simulink model "Quadcopter_FE_and_FTC_Sim"  (R2021a)
settings: Solver=VariableStepAuto  StartTime=0.0  StopTime=10.0  RelTol=1e-3
values from neighbouring files (symbols this model uses):
  A1_bar = [A1 E;zeros(3,6) zeros(3,3)]    [Quadcopter_Fault_Parameters_and_Flags.m]
  A2_bar = [A2 E;zeros(3,6) zeros(3,3)]    [Quadcopter_Fault_Parameters_and_Flags.m]
  A3_bar = [A3 E;zeros(3,6) zeros(3,3)]    [Quadcopter_Fault_Parameters_and_Flags.m]
  A4_bar = [A4 E;zeros(3,6) zeros(3,3)]    [Quadcopter_Fault_Parameters_and_Flags.m]
  B_bar = [B;zeros(3,3)]    [Quadcopter_Fault_Parameters_and_Flags.m]
  d = 0.0301    [Quadcopter_Fault_Parameters_and_Flags.m]
  Delta_q = [1 1 1 1;1 -1 -1 1;1 1 -1 -1;-1 1 -1 1]    [Quadcopter_Fault_Parameters_and_Flags.m]
  g = 9.8066    [Quadcopter_Fault_Parameters_and_Flags.m]
  Jrz = 2.029 * 10^(-5)    (= 2.029e-05)    [Quadcopter_Fault_Parameters_and_Flags.m]
  Jx = 0.0022    [Quadcopter_Fault_Parameters_and_Flags.m]
  Jy = 0.0029    [Quadcopter_Fault_Parameters_and_Flags.m]
  Jz = 0.0048    [Quadcopter_Fault_Parameters_and_Flags.m]
  K_D_kesi = diag([0.08,0.08,0.22])    [Quadcopter_Fault_Parameters_and_Flags.m]
  K_D_omega = diag([0.2,0.2,0.5])    [Quadcopter_Fault_Parameters_and_Flags.m]
  K_P_kesi = diag([0.18,0.18,052])    [Quadcopter_Fault_Parameters_and_Flags.m]
  K_P_omega = diag([1.5,1.5,2])    [Quadcopter_Fault_Parameters_and_Flags.m]
  kesi_d = [0 0 0]'    [Quadcopter_Fault_Parameters_and_Flags.m]
  kesi_dot_d = [0 0 0]'    [Quadcopter_Fault_Parameters_and_Flags.m]
  l = 0.1785    [Quadcopter_Fault_Parameters_and_Flags.m]
  LPI1_bar = (P^-1)*M    [Quadcopter_Fault_Parameters_and_Flags.m]
  LPI2_bar = (P^-1)*M    [Quadcopter_Fault_Parameters_and_Flags.m]
  LPI3_bar = (P^-1)*M    [Quadcopter_Fault_Parameters_and_Flags.m]
  LPI4_bar = (P^-1)*M    [Quadcopter_Fault_Parameters_and_Flags.m]
  m = 0.4080    (= 0.408)    [Quadcopter_Fault_Parameters_and_Flags.m]
  O_d = [0 0 0]'    [Quadcopter_Fault_Parameters_and_Flags.m]
  Omega_d = [0 0 0]'    [Quadcopter_Fault_Parameters_and_Flags.m]
  Omega_M = 475    [Quadcopter_Fault_Parameters_and_Flags.m]
  Phi_dot_init = 0    [Quadcopter_Fault_Parameters_and_Flags.m]
  Phi_init = 0    [Quadcopter_Fault_Parameters_and_Flags.m]
  Psi_dot_init = 0    [Quadcopter_Fault_Parameters_and_Flags.m]
  Psi_init = 0    [Quadcopter_Fault_Parameters_and_Flags.m]
  Theta_dot_init = 0    [Quadcopter_Fault_Parameters_and_Flags.m]
  Theta_init = 0    [Quadcopter_Fault_Parameters_and_Flags.m]
  x_dot_init = 0    [Quadcopter_Fault_Parameters_and_Flags.m]
  x_init = 0    [Quadcopter_Fault_Parameters_and_Flags.m]
  y_dot_init = 0    [Quadcopter_Fault_Parameters_and_Flags.m]
  y_init = 0    [Quadcopter_Fault_Parameters_and_Flags.m]
  z_dot_init = 0    [Quadcopter_Fault_Parameters_and_Flags.m]
  z_init = 0    [Quadcopter_Fault_Parameters_and_Flags.m]
settings Model: Creator=kiankhaneghahi  LastModifiedBy=kiankhaneghahi

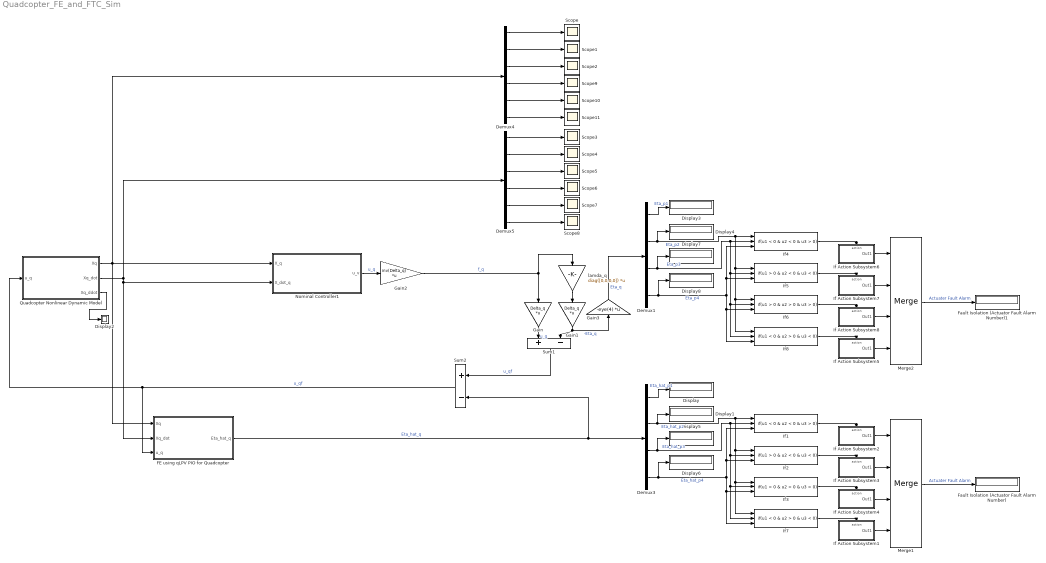
== system Quadcopter_FE_and_FTC_Sim ==
  Demux1 : Demux
  Demux3 : Demux
  Demux4 : Demux  Outputs=6
  Demux5 : Demux  Outputs=6
  Display{,1..8} (9 alike) : Display
  FE using qLPV PIO for Quadcopter : Subsystem
  Fault Isolation (Actuator Fault Alarm Number) : Display
  Fault Isolation (Actuator Fault Alarm Number)1 : Display
  Gain : Gain  Gain=Delta_q  Multiplication=Matrix(K*u)
  Gain1 : Gain  Gain=Delta_q  Multiplication=Matrix(K*u)
  Gain2 : Gain  Gain=inv(Delta_q)  Multiplication=Matrix(K*u)
  Gain3 : Gain  Gain=-eye(4)  Multiplication=Matrix(K*u)
  If Action Subsystem1 : Subsystem  TreatAsAtomicUnit=on
  If Action Subsystem2 : Subsystem  TreatAsAtomicUnit=on
  If Action Subsystem3 : Subsystem  TreatAsAtomicUnit=on
  If Action Subsystem4 : Subsystem  TreatAsAtomicUnit=on
  If Action Subsystem5 : Subsystem  TreatAsAtomicUnit=on
  If Action Subsystem6 : Subsystem  TreatAsAtomicUnit=on
  If Action Subsystem7 : Subsystem  TreatAsAtomicUnit=on
  If Action Subsystem8 : Subsystem  TreatAsAtomicUnit=on
  If1 : If  NumInputs=3  IfExpression=u1 < 0 & u2 < 0 & u3 > 0  ShowElse=off
  If2 : If  NumInputs=3  IfExpression=u1 > 0 & u2 < 0 & u3 < 0  ShowElse=off
  If3 : If  NumInputs=3  IfExpression=u1 > 0 & u2 > 0 & u3 > 0  ShowElse=off
  If4 : If  NumInputs=3  IfExpression=u1 < 0 & u2 < 0 & u3 > 0  ShowElse=off
  If5 : If  NumInputs=3  IfExpression=u1 > 0 & u2 < 0 & u3 < 0  ShowElse=off
  If6 : If  NumInputs=3  IfExpression=u1 > 0 & u2 > 0 & u3 > 0  ShowElse=off
  If7 : If  NumInputs=3  IfExpression=u1 < 0 & u2 > 0 & u3 < 0  ShowElse=off
  If8 : If  NumInputs=3  IfExpression=u1 < 0 & u2 > 0 & u3 < 0  ShowElse=off
  Merge1 : Merge  Inputs=4
  Merge2 : Merge  Inputs=4
  Nominal Controller1 : Subsystem
  Quadcopter Nonlinear Dynamic Model : Subsystem
  Scope{,1..11} (12 alike) : Scope
  Sum1 : Sum  Inputs=+-
  Sum2 : Sum  Inputs=+-
  lamda_q : Gain  Gain=diag([0,0,0,0])  Multiplication=Matrix(K*u)
  wires:
  If Action Subsystem3/1(Out1) -> Merge1/2
  lamda_q/1 -> Gain1/1
  Demux3/2 -> If7/1, If3/1, If2/1, If1/1, Display1/1  "Eta_hat_p2"
  Demux5/2 -> Scope4/1
  Demux3/3 -> If3/2, If7/2, If2/2, If1/2, Display5/1  "Eta_hat_p3"
  If2/1 -> If Action Subsystem3/Action
  Gain/1 -> Sum1/1  "u_q"
  Quadcopter Nonlinear Dynamic Model/2(Xq_dot) -> Demux5/1, Nominal Controller1/2(X_dot_q), FE using qLPV PIO for Quadcopter/2(Xq_dot)
  Merge1/1 -> Fault Isolation (Actuator Fault Alarm Number)/1  "Actuater Fault Alarm"
  If Action Subsystem4/1(Out1) -> Merge1/3
  If1/1 -> If Action Subsystem2/Action
  Demux4/1 -> Scope/1
  Nominal Controller1/1(u_v) -> Gain2/1  "u_q"
  Quadcopter Nonlinear Dynamic Model/1(Xq) -> Nominal Controller1/1(X_q), Demux4/1, FE using qLPV PIO for Quadcopter/1(Xq)
  Demux4/3 -> Scope2/1
  Demux4/2 -> Scope1/1
  Quadcopter Nonlinear Dynamic Model/3(Xq_ddot) -> Display2/1
  Gain2/1 -> Gain/1, lamda_q/1  "f_q"
  If Action Subsystem2/1(Out1) -> Merge1/1
  If3/1 -> If Action Subsystem4/Action
  Demux5/1 -> Scope3/1
  FE using qLPV PIO for Quadcopter/1(Eta_hat_q) -> Sum2/2, Demux3/1  "Eta_hat_q"
  Demux5/3 -> Scope5/1
  Sum2/1 -> Quadcopter Nonlinear Dynamic Model/1("u_q "), FE using qLPV PIO for Quadcopter/3(u_q)  "u_qf"
  Gain1/1 -> Sum1/2, Gain3/1  "-Eta_q"
  Gain3/1 -> Demux1/1  "Eta_q"
  Demux5/4 -> Scope6/1
  Demux5/5 -> Scope7/1
  Demux5/6 -> Scope8/1
  Demux4/5 -> Scope10/1
  Demux4/4 -> Scope9/1
  Demux4/6 -> Scope11/1
  Demux3/1 -> Display/1  "Eta_hat_p1"
  Demux3/4 -> If7/3, If3/3, If2/3, If1/3, Display6/1  "Eta_hat_p4"
  If Action Subsystem1/1(Out1) -> Merge1/4
  If7/1 -> If Action Subsystem1/Action
  Merge2/1 -> Fault Isolation (Actuator Fault Alarm Number)1/1  "Actuater Fault Alarm"
  If Action Subsystem8/1(Out1) -> Merge2/3
  If6/1 -> If Action Subsystem8/Action
  Demux1/1 -> Display3/1  "Eta_p1"
  If Action Subsystem7/1(Out1) -> Merge2/2
  If Action Subsystem6/1(Out1) -> Merge2/1
  If4/1 -> If Action Subsystem6/Action
  Demux1/3 -> If6/2, If8/2, If5/2, If4/2, Display7/1  "Eta_p3"
  Demux1/4 -> If8/3, If6/3, If5/3, If4/3, Display8/1  "Eta_p4"
  If5/1 -> If Action Subsystem7/Action
  Demux1/2 -> If8/1, If6/1, If5/1, If4/1, Display4/1  "Eta_p2"
  If8/1 -> If Action Subsystem5/Action
  If Action Subsystem5/1(Out1) -> Merge2/4
  Sum1/1 -> Sum2/1  "u_qf"

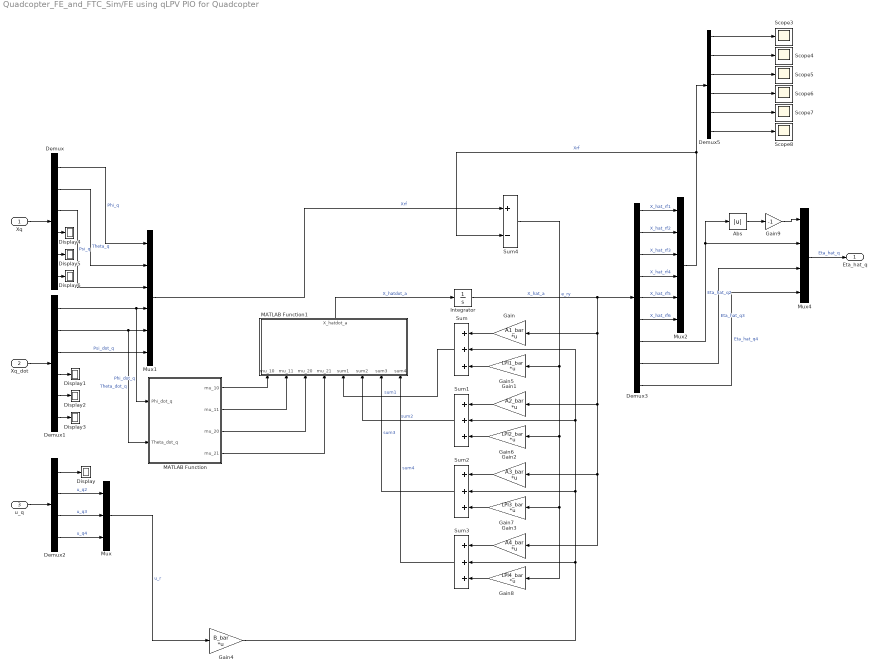
== system Quadcopter_FE_and_FTC_Sim/FE using qLPV PIO for Quadcopter ==
  Xq : Inport
  Xq_dot : Inport  Port=2
  u_q : Inport  Port=3
  Abs : Abs
  Demux : Demux  Outputs=6
  Demux1 : Demux  Outputs=6
  Demux2 : Demux
  Demux3 : Demux  Outputs=9
  Demux5 : Demux  Outputs=6
  Display{,1..6} (7 alike) : Display
  Gain : Gain  Gain=A1_bar  Multiplication=Matrix(K*u)
  Gain1 : Gain  Gain=A2_bar  Multiplication=Matrix(K*u)
  Gain2 : Gain  Gain=A3_bar  Multiplication=Matrix(K*u)
  Gain3 : Gain  Gain=A4_bar  Multiplication=Matrix(K*u)
  Gain4 : Gain  Gain=B_bar  Multiplication=Matrix(K*u)
  Gain5 : Gain  Gain=LPI1_bar  Multiplication=Matrix(K*u)
  Gain6 : Gain  Gain=LPI2_bar  Multiplication=Matrix(K*u)
  Gain7 : Gain  Gain=LPI3_bar  Multiplication=Matrix(K*u)
  Gain8 : Gain  Gain=LPI4_bar  Multiplication=Matrix(K*u)
  Gain9 : Gain  Gain=-1
  Integrator : Integrator
  MATLAB Function : MATLAB Function  TreatAsAtomicUnit=on
  MATLAB Function1 : MATLAB Function  TreatAsAtomicUnit=on
  Mux : Mux  Inputs=3
  Mux1 : Mux  Inputs=6
  Mux2 : Mux  Inputs=6
  Mux4 : Mux
  Scope{3..8} (6 alike) : Scope
  Sum{,1..3} (4 alike) : Sum  Inputs=+++
  Sum4 : Sum  Inputs=+-
  Eta_hat_q : Outport
  wires:
  Xq/1 -> Demux/1
  Xq_dot/1 -> Demux1/1
  u_q/1 -> Demux2/1
  Demux2/3 -> Mux/2  "u_q3"
  Demux2/2 -> Mux/1  "u_q2"
  Demux2/4 -> Mux/3  "u_q4"
  Mux/1 -> Gain4/1  "u_r"
  Demux/1 -> Mux1/1  "Phi_q"
  Demux/2 -> Mux1/2  "Theta_q"
  Demux/3 -> Mux1/3  "Psi_q"
  Demux1/1 -> MATLAB Function/1(Phi_dot_q), Mux1/4  "Phi_dot_q"
  Demux1/2 -> MATLAB Function/2(Theta_dot_q), Mux1/5  "Theta_dot_q"
  Demux1/3 -> Mux1/6  "Psi_dot_q"
  Mux1/1 -> Sum4/1  "Xrf"
  MATLAB Function1/1(X_hatdot_a) -> Integrator/1  "X_hatdot_a"
  Integrator/1 -> Gain3/1, Gain2/1, Gain1/1, Gain/1, Demux3/1  "X_hat_a"
  Gain/1 -> Sum/1
  Gain1/1 -> Sum1/1
  Gain2/1 -> Sum2/1
  Gain3/1 -> Sum3/1
  Gain4/1 -> Sum/2, Sum1/2, Sum2/2, Sum3/2
  Gain7/1 -> Sum2/3
  Gain5/1 -> Sum/3
  Gain6/1 -> Sum1/3
  Gain8/1 -> Sum3/3
  Demux3/1 -> Mux2/1  "X_hat_rf1"
  Demux3/2 -> Mux2/2  "X_hat_rf2"
  Demux3/3 -> Mux2/3  "X_hat_rf3"
  Demux3/4 -> Mux2/4  "X_hat_rf4"
  Demux3/5 -> Mux2/5  "X_hat_rf5"
  Demux3/6 -> Mux2/6  "X_hat_rf6"
  Demux3/7 -> Abs/1, Mux4/2  "Eta_hat_q2"
  Demux3/8 -> Mux4/3  "Eta_hat_q3"
  Demux3/9 -> Mux4/4  "Eta_hat_q4"
  Mux2/1 -> Demux5/1, Sum4/2  "Xrf"
  Sum4/1 -> Gain8/1, Gain7/1, Gain6/1, Gain5/1  "e_ry"
  Mux4/1 -> Eta_hat_q/1  "Eta_hat_q"
  Abs/1 -> Gain9/1
  Gain9/1 -> Mux4/1
  MATLAB Function/1(mu_10) -> MATLAB Function1/1(mu_10)
  MATLAB Function/2(mu_11) -> MATLAB Function1/2(mu_11)
  MATLAB Function/3(mu_20) -> MATLAB Function1/3(mu_20)
  MATLAB Function/4(mu_21) -> MATLAB Function1/4(mu_21)
  Sum/1 -> MATLAB Function1/5(sum1)  "sum1"
  Sum1/1 -> MATLAB Function1/6(sum2)  "sum2"
  Sum2/1 -> MATLAB Function1/7(sum3)  "sum3"
  Sum3/1 -> MATLAB Function1/8(sum4)  "sum4"
  Demux2/1 -> Display/1
  Demux1/4 -> Display1/1
  Demux1/5 -> Display2/1
  Demux1/6 -> Display3/1
  Demux/4 -> Display4/1
  Demux/5 -> Display5/1
  Demux/6 -> Display6/1
  Demux5/4 -> Scope6/1
  Demux5/1 -> Scope3/1
  Demux5/6 -> Scope8/1
  Demux5/2 -> Scope4/1
  Demux5/3 -> Scope5/1
  Demux5/5 -> Scope7/1

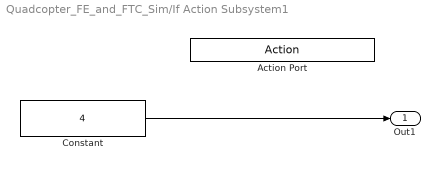
== system Quadcopter_FE_and_FTC_Sim/If Action Subsystem1 ==
  Action Port : ActionPort  ActionPortLabel=if(u1 < 0 & u2 > 0 & u3 < 0)
  Constant : Constant  Value=4
  Out1 : Outport
  wires:
  Constant/1 -> Out1/1

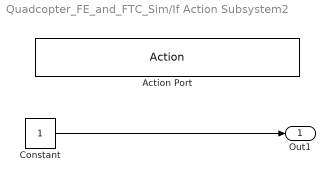
== system Quadcopter_FE_and_FTC_Sim/If Action Subsystem2 ==
  Action Port : ActionPort  ActionPortLabel=if(u1 < 0 & u2 < 0 & u3 > 0)
  Constant : Constant
  Out1 : Outport
  wires:
  Constant/1 -> Out1/1

== system Quadcopter_FE_and_FTC_Sim/If Action Subsystem3 ==
  Action Port : ActionPort  ActionPortLabel=if(u1 > 0 & u2 < 0 & u3 < 0)
  Constant : Constant  Value=2
  Out1 : Outport
  wires:
  Constant/1 -> Out1/1

== system Quadcopter_FE_and_FTC_Sim/If Action Subsystem4 ==
  Action Port : ActionPort  ActionPortLabel=if(u1 > 0 & u2 > 0 & u3 > 0)
  Constant : Constant  Value=3
  Out1 : Outport
  wires:
  Constant/1 -> Out1/1

== system Quadcopter_FE_and_FTC_Sim/If Action Subsystem5 ==
  Action Port : ActionPort  ActionPortLabel=if(u1 < 0 & u2 > 0 & u3 < 0)
  Constant : Constant  Value=4
  Out1 : Outport
  wires:
  Constant/1 -> Out1/1

== system Quadcopter_FE_and_FTC_Sim/If Action Subsystem6 ==
  Action Port : ActionPort  ActionPortLabel=if(u1 < 0 & u2 < 0 & u3 > 0)
  Constant : Constant
  Out1 : Outport
  wires:
  Constant/1 -> Out1/1

== system Quadcopter_FE_and_FTC_Sim/If Action Subsystem7 ==
  Action Port : ActionPort  ActionPortLabel=if(u1 > 0 & u2 < 0 & u3 < 0)
  Constant : Constant  Value=2
  Out1 : Outport
  wires:
  Constant/1 -> Out1/1

== system Quadcopter_FE_and_FTC_Sim/If Action Subsystem8 ==
  Action Port : ActionPort  ActionPortLabel=if(u1 > 0 & u2 > 0 & u3 > 0)
  Constant : Constant  Value=3
  Out1 : Outport
  wires:
  Constant/1 -> Out1/1

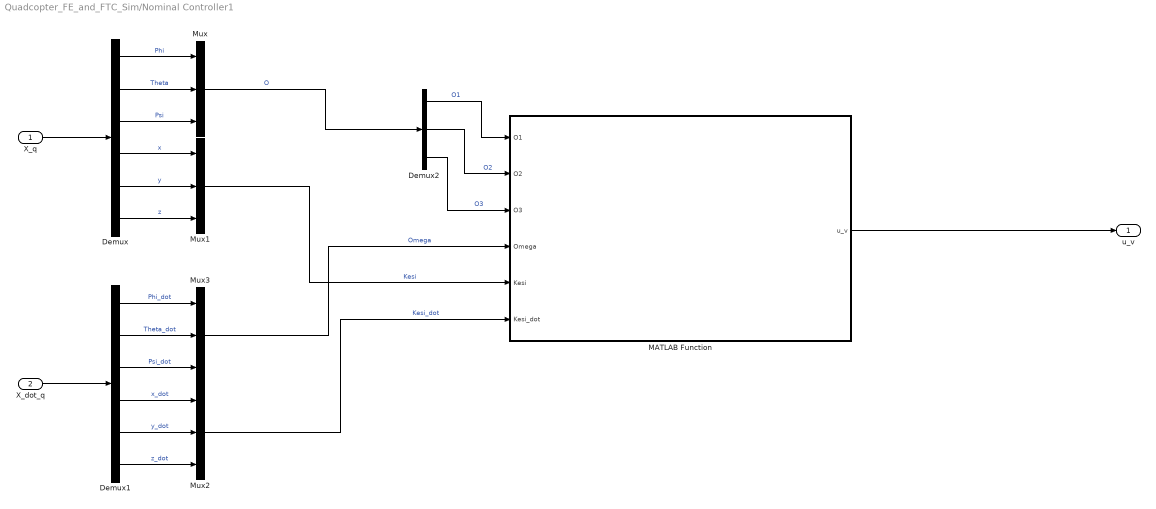
== system Quadcopter_FE_and_FTC_Sim/Nominal Controller1 ==
  X_q : Inport
  X_dot_q : Inport  Port=2
  Demux : Demux  Outputs=6
  Demux1 : Demux  Outputs=6
  Demux2 : Demux  Outputs=3
  MATLAB Function : MATLAB Function  TreatAsAtomicUnit=on
  Mux{,1..3} (4 alike) : Mux  Inputs=3
  u_v : Outport
  wires:
  X_q/1 -> Demux/1
  X_dot_q/1 -> Demux1/1
  Demux/3 -> Mux/3  "Psi"
  Demux/2 -> Mux/2  "Theta"
  Demux/1 -> Mux/1  "Phi"
  Demux/4 -> Mux1/1  "x"
  Demux/5 -> Mux1/2  "y"
  Demux/6 -> Mux1/3  "z"
  Demux1/4 -> Mux2/1  "x_dot"
  Demux1/5 -> Mux2/2  "y_dot"
  Demux1/6 -> Mux2/3  "z_dot"
  MATLAB Function/1(u_v) -> u_v/1
  Demux1/1 -> Mux3/1  "Phi_dot"
  Demux1/2 -> Mux3/2  "Theta_dot"
  Demux1/3 -> Mux3/3  "Psi_dot"
  Mux1/1 -> MATLAB Function/5(Kesi)  "Kesi"
  Mux2/1 -> MATLAB Function/6(Kesi_dot)  "Kesi_dot"
  Mux/1 -> Demux2/1  "O"
  Demux2/1 -> MATLAB Function/1(O1)  "O1"
  Demux2/2 -> MATLAB Function/2(O2)  "O2"
  Demux2/3 -> MATLAB Function/3(O3)  "O3"
  Mux3/1 -> MATLAB Function/4(Omega)  "Omega"

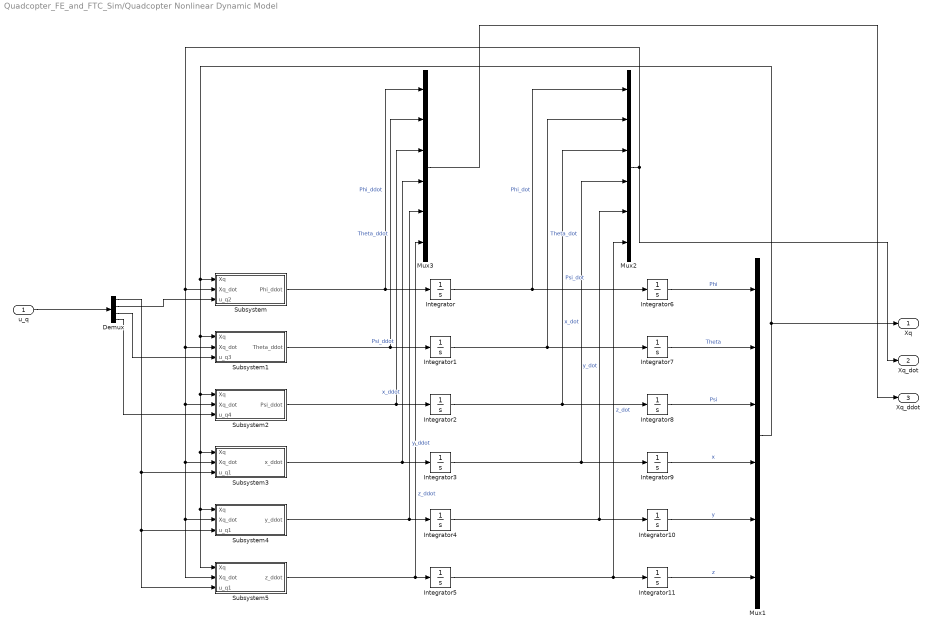
== system Quadcopter_FE_and_FTC_Sim/Quadcopter Nonlinear Dynamic Model ==
  "u_q " : Inport
  Demux : Demux
  Integrator : Integrator  InitialCondition=Phi_dot_init
  Integrator1 : Integrator  InitialCondition=Theta_dot_init
  Integrator10 : Integrator  InitialCondition=y_init
  Integrator11 : Integrator  InitialCondition=z_init
  Integrator2 : Integrator  InitialCondition=Psi_dot_init
  Integrator3 : Integrator  InitialCondition=x_dot_init
  Integrator4 : Integrator  InitialCondition=y_dot_init
  Integrator5 : Integrator  InitialCondition=z_dot_init
  Integrator6 : Integrator  InitialCondition=Phi_init
  Integrator7 : Integrator  InitialCondition=Theta_init
  Integrator8 : Integrator  InitialCondition=Psi_init
  Integrator9 : Integrator  InitialCondition=x_init
  Mux1 : Mux  Inputs=6
  Mux2 : Mux  Inputs=6
  Mux3 : Mux  Inputs=6
  Subsystem : Subsystem
  Subsystem1 : Subsystem
  Subsystem2 : Subsystem
  Subsystem3 : Subsystem
  Subsystem4 : Subsystem
  Subsystem5 : Subsystem
  Xq : Outport
  Xq_dot : Outport  Port=2
  Xq_ddot : Outport  Port=3
  wires:
  Integrator/1 -> Integrator6/1, Mux2/1  "Phi_dot"
  Integrator1/1 -> Mux2/2, Integrator7/1  "Theta_dot"
  Integrator2/1 -> Mux2/3, Integrator8/1  "Psi_dot"
  Integrator3/1 -> Mux2/4, Integrator9/1  "x_dot"
  Integrator4/1 -> Mux2/5, Integrator10/1  "y_dot"
  Integrator5/1 -> Mux2/6, Integrator11/1  "z_dot"
  Subsystem/1(Phi_ddot) -> Mux3/1, Integrator/1  "Phi_ddot"
  Subsystem5/1(z_ddot) -> Mux3/6, Integrator5/1  "z_ddot"
  Subsystem4/1(y_ddot) -> Mux3/5, Integrator4/1  "y_ddot"
  Subsystem3/1(x_ddot) -> Mux3/4, Integrator3/1  "x_ddot"
  Subsystem2/1(Psi_ddot) -> Mux3/3, Integrator2/1  "Psi_ddot"
  Subsystem1/1(Theta_ddot) -> Mux3/2, Integrator1/1  "Theta_ddot"
  "u_q "/1 -> Demux/1
  Demux/2 -> Subsystem/3(u_q2)
  Demux/3 -> Subsystem1/3(u_q3)
  Demux/4 -> Subsystem2/3(u_q4)
  Demux/1 -> Subsystem5/3(u_q1), Subsystem4/3(u_q1), Subsystem3/3(u_q1)
  Integrator6/1 -> Mux1/1  "Phi"
  Integrator7/1 -> Mux1/2  "Theta"
  Integrator8/1 -> Mux1/3  "Psi"
  Integrator9/1 -> Mux1/4  "x"
  Integrator10/1 -> Mux1/5  "y"
  Integrator11/1 -> Mux1/6  "z"
  Mux1/1 -> Subsystem5/1(Xq), Subsystem4/1(Xq), Subsystem3/1(Xq), Subsystem2/1(Xq), Subsystem1/1(Xq), Subsystem/1(Xq), Xq/1
  Mux2/1 -> Subsystem1/2(Xq_dot), Subsystem2/2(Xq_dot), Subsystem5/2(Xq_dot), Subsystem4/2(Xq_dot), Subsystem3/2(Xq_dot), Subsystem/2(Xq_dot), Xq_dot/1
  Mux3/1 -> Xq_ddot/1

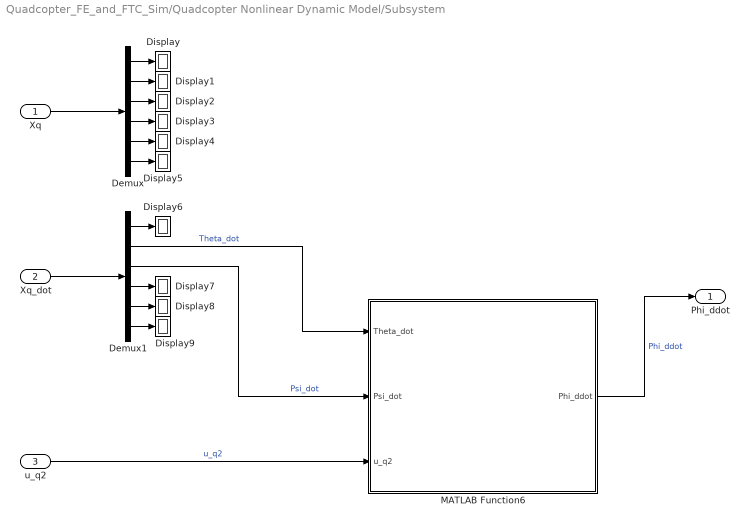
== system Quadcopter_FE_and_FTC_Sim/Quadcopter Nonlinear Dynamic Model/Subsystem ==
  Xq : Inport
  Xq_dot : Inport  Port=2
  u_q2 : Inport  Port=3
  Demux : Demux  Outputs=6
  Demux1 : Demux  Outputs=6
  Display{,1..9} (10 alike) : Display
  MATLAB Function6 : MATLAB Function  TreatAsAtomicUnit=on
  Phi_ddot : Outport
  wires:
  Xq/1 -> Demux/1
  Xq_dot/1 -> Demux1/1
  Demux1/2 -> MATLAB Function6/1(Theta_dot)  "Theta_dot"
  Demux1/3 -> MATLAB Function6/2(Psi_dot)  "Psi_dot"
  u_q2/1 -> MATLAB Function6/3(u_q2)  "u_q2"
  MATLAB Function6/1(Phi_ddot) -> Phi_ddot/1  "Phi_ddot"
  Demux/1 -> Display/1
  Demux/2 -> Display1/1
  Demux/3 -> Display2/1
  Demux/4 -> Display3/1
  Demux/5 -> Display4/1
  Demux/6 -> Display5/1
  Demux1/1 -> Display6/1
  Demux1/4 -> Display7/1
  Demux1/5 -> Display8/1
  Demux1/6 -> Display9/1

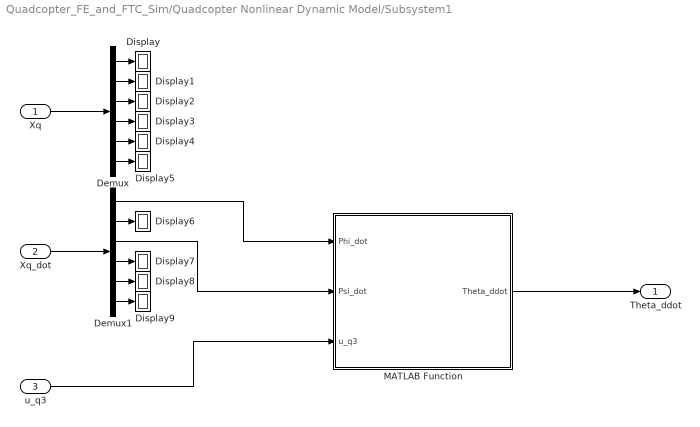
== system Quadcopter_FE_and_FTC_Sim/Quadcopter Nonlinear Dynamic Model/Subsystem1 ==
  Xq : Inport
  Xq_dot : Inport  Port=2
  u_q3 : Inport  Port=3
  Demux : Demux  Outputs=6
  Demux1 : Demux  Outputs=6
  Display{,1..9} (10 alike) : Display
  MATLAB Function : MATLAB Function  TreatAsAtomicUnit=on
  Theta_ddot : Outport
  wires:
  Xq/1 -> Demux/1
  Xq_dot/1 -> Demux1/1
  MATLAB Function/1(Theta_ddot) -> Theta_ddot/1
  u_q3/1 -> MATLAB Function/3(u_q3)
  Demux1/1 -> MATLAB Function/1(Phi_dot)
  Demux1/3 -> MATLAB Function/2(Psi_dot)
  Demux/1 -> Display/1
  Demux/2 -> Display1/1
  Demux/3 -> Display2/1
  Demux/4 -> Display3/1
  Demux/5 -> Display4/1
  Demux/6 -> Display5/1
  Demux1/2 -> Display6/1
  Demux1/4 -> Display7/1
  Demux1/5 -> Display8/1
  Demux1/6 -> Display9/1

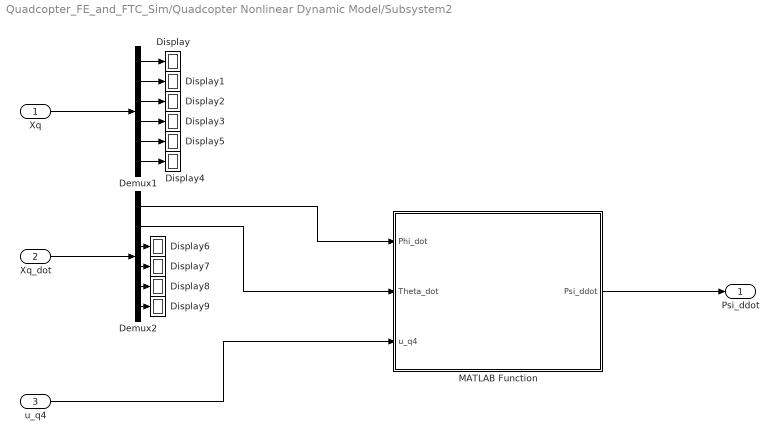
== system Quadcopter_FE_and_FTC_Sim/Quadcopter Nonlinear Dynamic Model/Subsystem2 ==
  Xq : Inport
  Xq_dot : Inport  Port=2
  u_q4 : Inport  Port=3
  Demux1 : Demux  Outputs=6
  Demux2 : Demux  Outputs=6
  Display{,1..9} (10 alike) : Display
  MATLAB Function : MATLAB Function  TreatAsAtomicUnit=on
  Psi_ddot : Outport
  wires:
  Xq/1 -> Demux1/1
  Xq_dot/1 -> Demux2/1
  MATLAB Function/1(Psi_ddot) -> Psi_ddot/1
  u_q4/1 -> MATLAB Function/3(u_q4)
  Demux2/1 -> MATLAB Function/1(Phi_dot)
  Demux2/2 -> MATLAB Function/2(Theta_dot)
  Demux1/1 -> Display/1
  Demux1/2 -> Display1/1
  Demux1/3 -> Display2/1
  Demux1/4 -> Display3/1
  Demux1/5 -> Display5/1
  Demux1/6 -> Display4/1
  Demux2/3 -> Display6/1
  Demux2/4 -> Display7/1
  Demux2/5 -> Display8/1
  Demux2/6 -> Display9/1

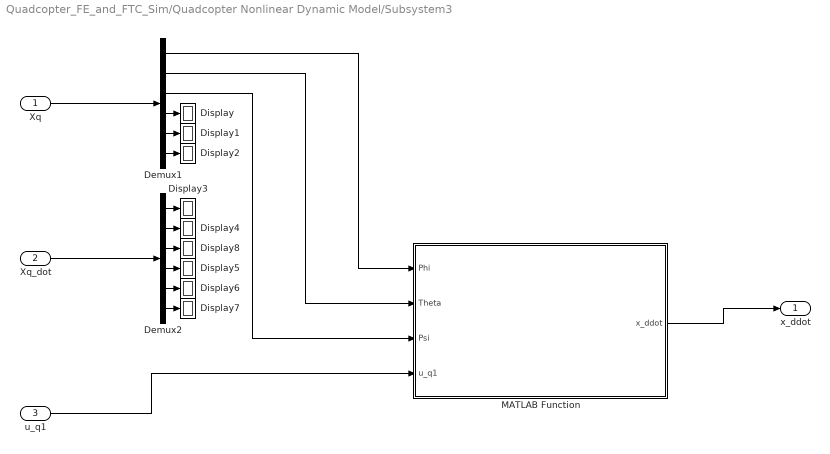
== system Quadcopter_FE_and_FTC_Sim/Quadcopter Nonlinear Dynamic Model/Subsystem3 ==
  Xq : Inport
  Xq_dot : Inport  Port=2
  u_q1 : Inport  Port=3
  Demux1 : Demux  Outputs=6
  Demux2 : Demux  Outputs=6
  Display{,1..8} (9 alike) : Display
  MATLAB Function : MATLAB Function  TreatAsAtomicUnit=on
  x_ddot : Outport
  wires:
  Xq/1 -> Demux1/1
  Xq_dot/1 -> Demux2/1
  MATLAB Function/1(x_ddot) -> x_ddot/1
  u_q1/1 -> MATLAB Function/4(u_q1)
  Demux1/1 -> MATLAB Function/1(Phi)
  Demux1/2 -> MATLAB Function/2(Theta)
  Demux1/3 -> MATLAB Function/3(Psi)
  Demux1/4 -> Display/1
  Demux1/5 -> Display1/1
  Demux1/6 -> Display2/1
  Demux2/1 -> Display3/1
  Demux2/2 -> Display4/1
  Demux2/3 -> Display8/1
  Demux2/4 -> Display5/1
  Demux2/5 -> Display6/1
  Demux2/6 -> Display7/1

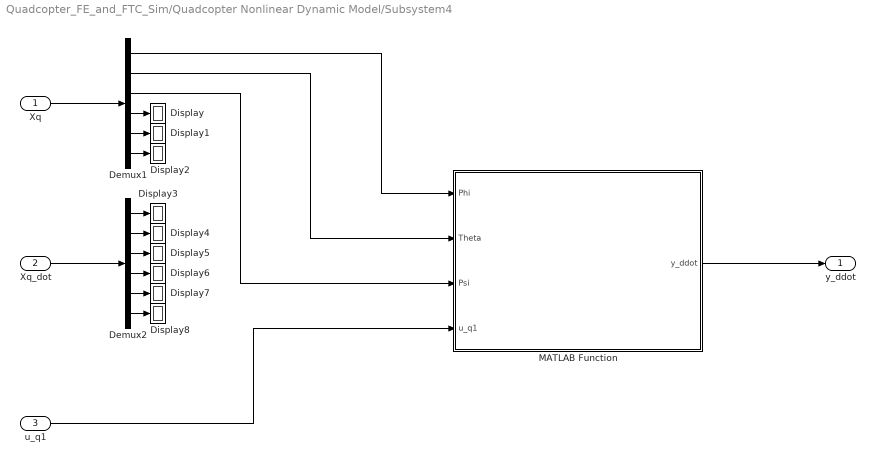
== system Quadcopter_FE_and_FTC_Sim/Quadcopter Nonlinear Dynamic Model/Subsystem4 ==
  Xq : Inport
  Xq_dot : Inport  Port=2
  u_q1 : Inport  Port=3
  Demux1 : Demux  Outputs=6
  Demux2 : Demux  Outputs=6
  Display{,1..8} (9 alike) : Display
  MATLAB Function : MATLAB Function  TreatAsAtomicUnit=on
  y_ddot : Outport
  wires:
  MATLAB Function/1(y_ddot) -> y_ddot/1
  Xq_dot/1 -> Demux2/1
  Xq/1 -> Demux1/1
  u_q1/1 -> MATLAB Function/4(u_q1)
  Demux1/1 -> MATLAB Function/1(Phi)
  Demux1/2 -> MATLAB Function/2(Theta)
  Demux1/3 -> MATLAB Function/3(Psi)
  Demux1/4 -> Display/1
  Demux1/5 -> Display1/1
  Demux1/6 -> Display2/1
  Demux2/1 -> Display3/1
  Demux2/2 -> Display4/1
  Demux2/3 -> Display5/1
  Demux2/4 -> Display6/1
  Demux2/5 -> Display7/1
  Demux2/6 -> Display8/1

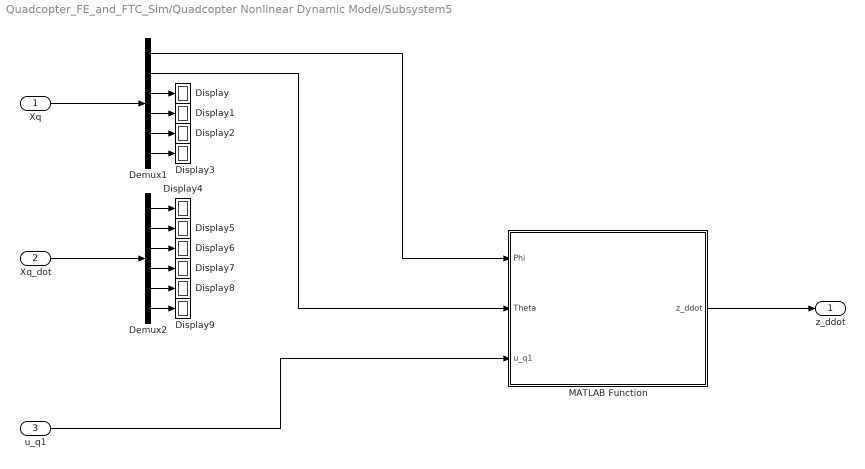
== system Quadcopter_FE_and_FTC_Sim/Quadcopter Nonlinear Dynamic Model/Subsystem5 ==
  Xq : Inport
  Xq_dot : Inport  Port=2
  u_q1 : Inport  Port=3
  Demux1 : Demux  Outputs=6
  Demux2 : Demux  Outputs=6
  Display{,1..9} (10 alike) : Display
  MATLAB Function : MATLAB Function  TreatAsAtomicUnit=on
  z_ddot : Outport
  wires:
  Xq/1 -> Demux1/1
  Xq_dot/1 -> Demux2/1
  MATLAB Function/1(z_ddot) -> z_ddot/1
  u_q1/1 -> MATLAB Function/3(u_q1)
  Demux1/1 -> MATLAB Function/1(Phi)
  Demux1/2 -> MATLAB Function/2(Theta)
  Demux1/3 -> Display/1
  Demux1/4 -> Display1/1
  Demux1/5 -> Display2/1
  Demux1/6 -> Display3/1
  Demux2/1 -> Display4/1
  Demux2/2 -> Display5/1
  Demux2/3 -> Display6/1
  Demux2/4 -> Display7/1
  Demux2/5 -> Display8/1
  Demux2/6 -> Display9/1

== matlab function Quadcopter_FE_and_FTC_Sim/FE using qLPV PIO for Quadcopter/MATLAB Function ==
  data: Phi_dot_q input; mu_10 output; Theta_dot_q input; mu_11 output; mu_20 output; mu_21 output
function [mu_10,mu_11,mu_20,mu_21] = fcn(Phi_dot_q, Theta_dot_q)
mu_10 = (pi-2*Phi_dot_q)/(2*pi);
mu_11 = 1-mu_10;
mu_20 = (pi-2*Theta_dot_q)/(2*pi);
mu_21 = 1-mu_20;

== matlab function Quadcopter_FE_and_FTC_Sim/FE using qLPV PIO for Quadcopter/MATLAB Function1 ==
  data: mu_10 input; X_hatdot_a output; mu_11 input; mu_20 input; mu_21 input; sum1 input; sum2 input; sum3 input; sum4 input
function X_hatdot_a = fcn(mu_10, mu_11, mu_20, mu_21, sum1, sum2, sum3, sum4)
ro_1 = mu_10 * mu_20;
ro_2 = mu_10 * mu_21;
ro_3 = mu_11 * mu_20;
ro_4 = mu_11 * mu_21;
X_hatdot_a = ro_1*sum1 + ro_2*sum2 + ro_3*sum3 + ro_4*sum4;

== matlab function Quadcopter_FE_and_FTC_Sim/Quadcopter Nonlinear Dynamic Model/Subsystem/MATLAB Function6 ==
  data: Theta_dot input; Phi_ddot output; Psi_dot input; u_q2 input; Jx parameter; Jy parameter; Jz parameter; Jrz parameter; Omega_M parameter; l parameter
function Phi_ddot = fcn(Theta_dot, Psi_dot, u_q2, Jx, Jy, Jz, Jrz, Omega_M, l)

Phi_ddot = Theta_dot*Psi_dot*((Jy-Jz)/Jx)-(Jrz/Jx)*Theta_dot*Omega_M+(l/Jx)*u_q2;

== matlab function Quadcopter_FE_and_FTC_Sim/Quadcopter Nonlinear Dynamic Model/Subsystem1/MATLAB Function ==
  data: Phi_dot input; Psi_dot input; u_q3 input; Theta_ddot output; Jx parameter; Jy parameter; Jz parameter; Jrz parameter; Omega_M parameter; l parameter
function Theta_ddot = fcn(Phi_dot, Psi_dot, u_q3, Jx, Jy, Jz, Jrz, Omega_M, l)

Theta_ddot = Phi_dot*Psi_dot*((Jz-Jx)/Jy)+(Jrz/Jy)*Phi_dot*Omega_M+(l/Jy)*u_q3;

== matlab function Quadcopter_FE_and_FTC_Sim/Quadcopter Nonlinear Dynamic Model/Subsystem2/MATLAB Function ==
  data: Phi_dot input; Theta_dot input; u_q4 input; Psi_ddot output; Jx parameter; Jy parameter; Jz parameter; d parameter
function Psi_ddot = fcn(Phi_dot, Theta_dot, u_q4, Jx, Jy, Jz, d)

Psi_ddot = Phi_dot*Theta_dot*((Jx-Jy)/Jz)+(d/Jz)*u_q4;

== matlab function Quadcopter_FE_and_FTC_Sim/Quadcopter Nonlinear Dynamic Model/Subsystem3/MATLAB Function ==
  data: Phi input; Theta input; Psi input; u_q1 input; x_ddot output; m parameter
function x_ddot = fcn(Phi, Theta, Psi, u_q1, m)

x_ddot = (cos(Psi)*sin(Theta)*cos(Phi)+sin(Psi)*sin(Phi))*(1/m)*u_q1;

== matlab function Quadcopter_FE_and_FTC_Sim/Quadcopter Nonlinear Dynamic Model/Subsystem4/MATLAB Function ==
  data: Phi input; Theta input; Psi input; u_q1 input; y_ddot output; m parameter
function y_ddot = fcn(Phi, Theta, Psi, u_q1, m)

y_ddot = (sin(Psi)*sin(Theta)*cos(Phi)-cos(Psi)*sin(Phi))*(1/m)*u_q1;

== matlab function Quadcopter_FE_and_FTC_Sim/Quadcopter Nonlinear Dynamic Model/Subsystem5/MATLAB Function ==
  data: Phi input; Theta input; u_q1 input; z_ddot output; g parameter; m parameter
function z_ddot = fcn(Phi, Theta, u_q1, g, m)

z_ddot = -g + cos(Theta)*cos(Phi)*(1/m)*u_q1;

== matlab function Quadcopter_FE_and_FTC_Sim/Nominal Controller1/MATLAB Function ==
  data: O1 input; O2 input; O3 input; Omega input; u_v output; Kesi input; Kesi_dot input; K_P_kesi parameter; kesi_d parameter; K_D_kesi parameter; kesi_dot_d parameter; K_P_omega parameter; K_D_omega parameter; Omega_d parameter; O_d parameter
function u_v = fcn(O1, O2, O3, Omega, Kesi, Kesi_dot, K_P_kesi, kesi_d, K_D_kesi, kesi_dot_d, K_P_omega, K_D_omega, Omega_d, O_d)
O = [O1,O2,O3]';
q = quaternion(O','euler','xyz','frame');
q_d = quaternion(O_d','euler','xyz','frame');
q_d_conj = conj(q_d);
q_e = q * q_d_conj;
%q_e_ln = 2*log(q_e);
q_e_eu = euler(q_e,'xyz','frame')';
u_v = [norm(-K_P_kesi*(Kesi-kesi_d)-K_D_kesi*(Kesi_dot-kesi_dot_d));-K_P_omega*q_e_eu-K_D_omega*(Omega-Omega_d)];
